simulink model "REL"  (R2022a)
settings: Solver=FixedStepDiscrete  StartTime=0.0  StopTime=10.0  FixedStep=0.01  RelTol=1e-3
libraries: simulink x4, DoorRatSts x4, DoorRlsDriver x4, DoorRlsReq x4
(part 1 of 2)
settings Model: Creator=DELL  LastModifiedBy=DELL
settings DataIOCC: SaveFormat=StructureWithTime
settings OptimizationCC: DefaultParameterBehavior=Inlined  EnhancedBackFolding=on  PassReuseOutputArgsAs=Individual arguments  ZeroExternalMemoryAtStartup=off  ZeroInternalMemoryAtStartup=off  OptimizeBlockOrder=speed  DifferentSizesBufferReuse=on  OptimizationCustomize=off  EfficientTunableParamExpr=on
settings DebuggingCC: ParameterTunabilityLossMsg=error
settings ModelReferenceCC: ModelReferenceNumInstancesAllowed=Single
settings SFSimCC: MATLABDynamicMemAlloc=off
settings RTWCC: SystemTargetFile=ert.tlc  GenCodeOnly=on  TemplateMakefile=ert_default_tmf
settings CodeAppCC: ForceParamTrailComments=on  IgnoreCustomStorageClasses=off  OperatorAnnotations=on  SimulinkDataObjDesc=on  SFDataObjDesc=on  InsertBlockDesc=on
settings ERTTargetCC: TargetLangStandard=C99 (ISO)  GenerateSampleERTMain=on  InlinedParameterPlacement=NonHierarchical  ERTCustomFileTemplate=example_file_process.tlc

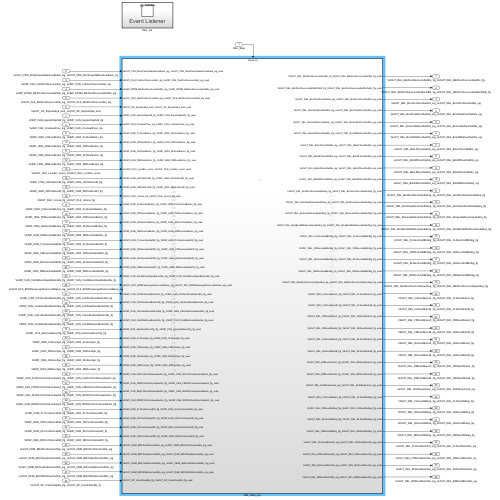
[thumbnail: Simulink's stored preview of the top-level diagram]
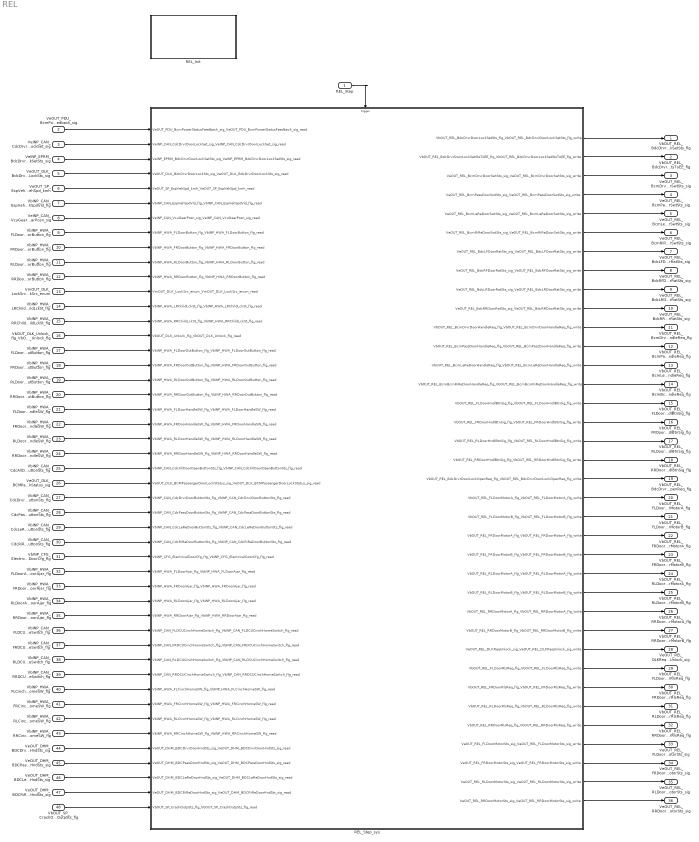
== system REL ==
  REL_Step : Inport  SampleTime=0.01  OutputFunctionCall=on
  VeOUT_PDU_BcmPowerStatusFeedback_sig_VeOUT_PDU_BcmPowerStatusFeedback_sig : Inport  Port=2  OutDataTypeStr=UInt8  PortDimensions=1
  VeINP_CAN_CdcDrvrDoorLockSet_sig_VeINP_CAN_CdcDrvrDoorLockSet_sig : Inport  Port=3  OutDataTypeStr=UInt8  PortDimensions=1
  VeINP_EPRM_BdcDrvrDoorLockSetSts_sig_VeINP_EPRM_BdcDrvrDoorLockSetSts_sig : Inport  Port=4  OutDataTypeStr=UInt8  PortDimensions=1
  VeOUT_DLK_BdcDrvrDoorLockSts_sig_VeOUT_DLK_BdcDrvrDoorLockSts_sig : Inport  Port=5  OutDataTypeStr=UInt8  PortDimensions=1
  VeOUT_SP_EspVehSpd_kmh_VeOUT_SP_EspVehSpd_kmh : Inport  Port=6  OutDataTypeStr=UInt8  PortDimensions=1
  VbINP_CAN_EspVehSpdVld_flg_VbINP_CAN_EspVehSpdVld_flg : Inport  Port=7  OutDataTypeStr=Boolean  PortDimensions=1
  VeINP_CAN_VcuGearPosn_sig_VeINP_CAN_VcuGearPosn_sig : Inport  Port=8  OutDataTypeStr=UInt8  PortDimensions=1
  VbINP_HWA_FLDoorButton_flg_VbINP_HWA_FLDoorButton_flg : Inport  Port=9  OutDataTypeStr=Boolean  PortDimensions=1
  VbINP_HWA_FRDoorButton_flg_VbINP_HWA_FRDoorButton_flg : Inport  Port=10  OutDataTypeStr=Boolean  PortDimensions=1
  VbINP_HWA_RLDoorButton_flg_VbINP_HWA_RLDoorButton_flg : Inport  Port=11  OutDataTypeStr=Boolean  PortDimensions=1
  VbINP_HWA_RRDoorButton_flg_VbINP_HWA_RRDoorButton_flg : Inport  Port=12  OutDataTypeStr=Boolean  PortDimensions=1
  VmOUT_DLK_LockSrc_enum_VmOUT_DLK_LockSrc_enum : Inport  Port=13  OutDataTypeStr=UInt8  PortDimensions=1
  VbINP_HWA_LRChildLckSt_flg_VbINP_HWA_LRChildLckSt_flg : Inport  Port=14  OutDataTypeStr=Boolean  PortDimensions=1
  VbINP_HWA_RRChildLckSt_flg_VbINP_HWA_RRChildLckSt_flg : Inport  Port=15  OutDataTypeStr=Boolean  PortDimensions=1
  VbOUT_DLK_Unlock_flg_VbOUT_DLK_Unlock_flg : Inport  Port=16  OutDataTypeStr=Boolean  PortDimensions=1
  VbINP_HWA_FLDoorOutButton_flg_VbINP_HWA_FLDoorOutButton_flg : Inport  Port=17  OutDataTypeStr=Boolean  PortDimensions=1
  VbINP_HWA_FRDoorOutButton_flg_VbINP_HWA_FRDoorOutButton_flg : Inport  Port=18  OutDataTypeStr=Boolean  PortDimensions=1
  VbINP_HWA_RLDoorOutButton_flg_VbINP_HWA_RLDoorOutButton_flg : Inport  Port=19  OutDataTypeStr=Boolean  PortDimensions=1
  VbINP_HWA_RRDoorOutButton_flg_VbINP_HWA_RRDoorOutButton_flg : Inport  Port=20  OutDataTypeStr=Boolean  PortDimensions=1
  VbINP_HWA_FLDoorHandleSW_flg_VbINP_HWA_FLDoorHandleSW_flg : Inport  Port=21  OutDataTypeStr=Boolean  PortDimensions=1
  VbINP_HWA_FRDoorHandleSW_flg_VbINP_HWA_FRDoorHandleSW_flg : Inport  Port=22  OutDataTypeStr=Boolean  PortDimensions=1
  VbINP_HWA_RLDoorHandleSW_flg_VbINP_HWA_RLDoorHandleSW_flg : Inport  Port=23  OutDataTypeStr=Boolean  PortDimensions=1
  VbINP_HWA_RRDoorHandleSW_flg_VbINP_HWA_RRDoorHandleSW_flg : Inport  Port=24  OutDataTypeStr=Boolean  PortDimensions=1
  VbINP_CAN_CdcAllDoorOpenButtonSts_flg_VbINP_CAN_CdcAllDoorOpenButtonSts_flg : Inport  Port=25  OutDataTypeStr=Boolean  PortDimensions=1
  VeOUT_DLK_BCMPassengerDoorLockStatus_sig_VeOUT_DLK_BCMPassengerDoorLockStatus_sig : Inport  Port=26  OutDataTypeStr=UInt8  PortDimensions=1
  VbINP_CAN_CdcDrvrDoorButtonSts_flg_VbINP_CAN_CdcDrvrDoorButtonSts_flg : Inport  Port=27  OutDataTypeStr=Boolean  PortDimensions=1
  VbINP_CAN_CdcPassDoorButtonSts_flg_VbINP_CAN_CdcPassDoorButtonSts_flg : Inport  Port=28  OutDataTypeStr=Boolean  PortDimensions=1
  VbINP_CAN_CdcLeReDoorButtonSts_flg_VbINP_CAN_CdcLeReDoorButtonSts_flg : Inport  Port=29  OutDataTypeStr=Boolean  PortDimensions=1
  VbINP_CAN_CdcRiReDoorButtonSts_flg_VbINP_CAN_CdcRiReDoorButtonSts_flg : Inport  Port=30  OutDataTypeStr=Boolean  PortDimensions=1
  VbINP_CFG_ElectricalDoorCfg_flg_VbINP_CFG_ElectricalDoorCfg_flg : Inport  Port=31  OutDataTypeStr=Boolean  PortDimensions=1
  VbINP_HWA_FLDoorAjar_flg_VbINP_HWA_FLDoorAjar_flg : Inport  Port=32  OutDataTypeStr=Boolean  PortDimensions=1
  VbINP_HWA_FRDoorAjar_flg_VbINP_HWA_FRDoorAjar_flg : Inport  Port=33  OutDataTypeStr=Boolean  PortDimensions=1
  VbINP_HWA_RLDoorAjar_flg_VbINP_HWA_RLDoorAjar_flg : Inport  Port=34  OutDataTypeStr=Boolean  PortDimensions=1
  VbINP_HWA_RRDoorAjar_flg_VbINP_HWA_RRDoorAjar_flg : Inport  Port=35  OutDataTypeStr=Boolean  PortDimensions=1
  VbINP_CAN_FLDCUCinchHomeSwitch_flg_VbINP_CAN_FLDCUCinchHomeSwitch_flg : Inport  Port=36  OutDataTypeStr=Boolean  PortDimensions=1
  VbINP_CAN_FRDCUCinchHomeSwitch_flg_VbINP_CAN_FRDCUCinchHomeSwitch_flg : Inport  Port=37  OutDataTypeStr=Boolean  PortDimensions=1
  VbINP_CAN_RLDCUCinchHomeSwitch_flg_VbINP_CAN_RLDCUCinchHomeSwitch_flg : Inport  Port=38  OutDataTypeStr=Boolean  PortDimensions=1
  VbINP_CAN_RRDCUCinchHomeSwitch_flg_VbINP_CAN_RRDCUCinchHomeSwitch_flg : Inport  Port=39  OutDataTypeStr=Boolean  PortDimensions=1
  VbINP_HWA_FLCinchHomeSW_flg_VbINP_HWA_FLCinchHomeSW_flg : Inport  Port=40  OutDataTypeStr=Boolean  PortDimensions=1
  VbINP_HWA_FRCinchHomeSW_flg_VbINP_HWA_FRCinchHomeSW_flg : Inport  Port=41  OutDataTypeStr=Boolean  PortDimensions=1
  VbINP_HWA_RLCinchHomeSW_flg_VbINP_HWA_RLCinchHomeSW_flg : Inport  Port=42  OutDataTypeStr=Boolean  PortDimensions=1
  VbINP_HWA_RRCinchHomeSW_flg_VbINP_HWA_RRCinchHomeSW_flg : Inport  Port=43  OutDataTypeStr=Boolean  PortDimensions=1
  VeOUT_DHM_BDCDrvrDoorHndSts_sig_VeOUT_DHM_BDCDrvrDoorHndSts_sig : Inport  Port=44  OutDataTypeStr=UInt8  PortDimensions=1
  VeOUT_DHM_BDCPassDoorHndSts_sig_VeOUT_DHM_BDCPassDoorHndSts_sig : Inport  Port=45  OutDataTypeStr=UInt8  PortDimensions=1
  VeOUT_DHM_BDCLeReDoorHndSts_sig_VeOUT_DHM_BDCLeReDoorHndSts_sig : Inport  Port=46  OutDataTypeStr=UInt8  PortDimensions=1
  VeOUT_DHM_BDCRiReDoorHndSts_sig_VeOUT_DHM_BDCRiReDoorHndSts_sig : Inport  Port=47  OutDataTypeStr=UInt8  PortDimensions=1
  VbOUT_SP_CrashOutpSts_flg_VbOUT_SP_CrashOutpSts_flg : Inport  Port=48  OutDataTypeStr=Boolean  PortDimensions=1
  REL_Init : Subsystem
  REL_Step_sys : Subsystem
  VbOUT_REL_BdcDrvrDoorLockSetSts_flg_VbOUT_REL_BdcDrvrDoorLockSetSts_flg : Outport  OutDataTypeStr=Boolean  PortDimensions=1
  VbOUT_REL_BdcDrvrDoorLockSetStsToEE_flg_VbOUT_REL_BdcDrvrDoorLockSetStsToEE_flg : Outport  Port=2  OutDataTypeStr=Boolean  PortDimensions=1
  VeOUT_REL_BcmDrvrDoorSwtSts_sig_VeOUT_REL_BcmDrvrDoorSwtSts_sig : Outport  Port=3  OutDataTypeStr=UInt8  PortDimensions=1
  VeOUT_REL_BcmPassDoorSwtSts_sig_VeOUT_REL_BcmPassDoorSwtSts_sig : Outport  Port=4  OutDataTypeStr=UInt8  PortDimensions=1
  VeOUT_REL_BcmLeReDoorSwtSts_sig_VeOUT_REL_BcmLeReDoorSwtSts_sig : Outport  Port=5  OutDataTypeStr=UInt8  PortDimensions=1
  VeOUT_REL_BcmRiReDoorSwtSts_sig_VeOUT_REL_BcmRiReDoorSwtSts_sig : Outport  Port=6  OutDataTypeStr=UInt8  PortDimensions=1
  VeOUT_REL_BdcLFDoorRatSts_sig_VeOUT_REL_BdcLFDoorRatSts_sig : Outport  Port=7  OutDataTypeStr=UInt8  PortDimensions=1
  VeOUT_REL_BdcRFDoorRatSts_sig_VeOUT_REL_BdcRFDoorRatSts_sig : Outport  Port=8  OutDataTypeStr=UInt8  PortDimensions=1
  VeOUT_REL_BdcLRDoorRatSts_sig_VeOUT_REL_BdcLRDoorRatSts_sig : Outport  Port=9  OutDataTypeStr=UInt8  PortDimensions=1
  VeOUT_REL_BdcRRDoorRatSts_sig_VeOUT_REL_BdcRRDoorRatSts_sig : Outport  Port=10  OutDataTypeStr=UInt8  PortDimensions=1
  VbOUT_REL_BcmDrvrDoorHandleReq_flg_VbOUT_REL_BcmDrvrDoorHandleReq_flg : Outport  Port=11  OutDataTypeStr=Boolean  PortDimensions=1
  VbOUT_REL_BcmPassDoorHandleReq_flg_VbOUT_REL_BcmPassDoorHandleReq_flg : Outport  Port=12  OutDataTypeStr=Boolean  PortDimensions=1
  VbOUT_REL_BcmLeReDoorHandleReq_flg_VbOUT_REL_BcmLeReDoorHandleReq_flg : Outport  Port=13  OutDataTypeStr=Boolean  PortDimensions=1
  VbOUT_REL_BcmBcmRiReDoorHandleReq_flg_VbOUT_REL_BcmBcmRiReDoorHandleReq_flg : Outport  Port=14  OutDataTypeStr=Boolean  PortDimensions=1
  VbOUT_REL_FLDoorHndlBtnSig_flg_VbOUT_REL_FLDoorHndlBtnSig_flg : Outport  Port=15  OutDataTypeStr=Boolean  PortDimensions=1
  VbOUT_REL_FRDoorHndlBtnSig_flg_VbOUT_REL_FRDoorHndlBtnSig_flg : Outport  Port=16  OutDataTypeStr=Boolean  PortDimensions=1
  VbOUT_REL_RLDoorHndlBtnSig_flg_VbOUT_REL_RLDoorHndlBtnSig_flg : Outport  Port=17  OutDataTypeStr=Boolean  PortDimensions=1
  VbOUT_REL_RRDoorHndlBtnSig_flg_VbOUT_REL_RRDoorHndlBtnSig_flg : Outport  Port=18  OutDataTypeStr=Boolean  PortDimensions=1
  VbOUT_REL_BdcDrvrDoorLockOpenReq_flg_VbOUT_REL_BdcDrvrDoorLockOpenReq_flg : Outport  Port=19  OutDataTypeStr=Boolean  PortDimensions=1
  VbOUT_REL_FLDoorMotorA_flg_VbOUT_REL_FLDoorMotorA_flg : Outport  Port=20  OutDataTypeStr=Boolean  PortDimensions=1
  VbOUT_REL_FLDoorMotorB_flg_VbOUT_REL_FLDoorMotorB_flg : Outport  Port=21  OutDataTypeStr=Boolean  PortDimensions=1
  VbOUT_REL_FRDoorMotorA_flg_VbOUT_REL_FRDoorMotorA_flg : Outport  Port=22  OutDataTypeStr=Boolean  PortDimensions=1
  VbOUT_REL_FRDoorMotorB_flg_VbOUT_REL_FRDoorMotorB_flg : Outport  Port=23  OutDataTypeStr=Boolean  PortDimensions=1
  VbOUT_REL_RLDoorMotorA_flg_VbOUT_REL_RLDoorMotorA_flg : Outport  Port=24  OutDataTypeStr=Boolean  PortDimensions=1
  VbOUT_REL_RLDoorMotorB_flg_VbOUT_REL_RLDoorMotorB_flg : Outport  Port=25  OutDataTypeStr=Boolean  PortDimensions=1
  VbOUT_REL_RRDoorMotorA_flg_VbOUT_REL_RRDoorMotorA_flg : Outport  Port=26  OutDataTypeStr=Boolean  PortDimensions=1
  VbOUT_REL_RRDoorMotorB_flg_VbOUT_REL_RRDoorMotorB_flg : Outport  Port=27  OutDataTypeStr=Boolean  PortDimensions=1
  VeOUT_REL_DLKReqUnlock_sig_VeOUT_REL_DLKReqUnlock_sig : Outport  Port=28  OutDataTypeStr=UInt8  PortDimensions=1
  VbOUT_REL_FLDoorRlsReq_flg_VbOUT_REL_FLDoorRlsReq_flg : Outport  Port=29  OutDataTypeStr=Boolean  PortDimensions=1
  VbOUT_REL_FRDoorRlsReq_flg_VbOUT_REL_FRDoorRlsReq_flg : Outport  Port=30  OutDataTypeStr=Boolean  PortDimensions=1
  VbOUT_REL_RLDoorRlsReq_flg_VbOUT_REL_RLDoorRlsReq_flg : Outport  Port=31  OutDataTypeStr=Boolean  PortDimensions=1
  VbOUT_REL_RRDoorRlsReq_flg_VbOUT_REL_RRDoorRlsReq_flg : Outport  Port=32  OutDataTypeStr=Boolean  PortDimensions=1
  VeOUT_REL_FLDoorMotorSts_sig_VeOUT_REL_FLDoorMotorSts_sig : Outport  Port=33  OutDataTypeStr=UInt8  PortDimensions=1
  VeOUT_REL_FRDoorMotorSts_sig_VeOUT_REL_FRDoorMotorSts_sig : Outport  Port=34  OutDataTypeStr=UInt8  PortDimensions=1
  VeOUT_REL_RLDoorMotorSts_sig_VeOUT_REL_RLDoorMotorSts_sig : Outport  Port=35  OutDataTypeStr=UInt8  PortDimensions=1
  VeOUT_REL_RRDoorMotorSts_sig_VeOUT_REL_RRDoorMotorSts_sig : Outport  Port=36  OutDataTypeStr=UInt8  PortDimensions=1
  wires:
  VeOUT_PDU_BcmPowerStatusFeedback_sig_VeOUT_PDU_BcmPowerStatusFeedback_sig/1 -> REL_Step_sys/1(VeOUT_PDU_BcmPowerStatusFeedback_sig_VeOUT_PDU_BcmPowerStatusFeedback_sig_read)
  VeINP_CAN_CdcDrvrDoorLockSet_sig_VeINP_CAN_CdcDrvrDoorLockSet_sig/1 -> REL_Step_sys/2(VeINP_CAN_CdcDrvrDoorLockSet_sig_VeINP_CAN_CdcDrvrDoorLockSet_sig_read)
  VeINP_EPRM_BdcDrvrDoorLockSetSts_sig_VeINP_EPRM_BdcDrvrDoorLockSetSts_sig/1 -> REL_Step_sys/3(VeINP_EPRM_BdcDrvrDoorLockSetSts_sig_VeINP_EPRM_BdcDrvrDoorLockSetSts_sig_read)
  VeOUT_DLK_BdcDrvrDoorLockSts_sig_VeOUT_DLK_BdcDrvrDoorLockSts_sig/1 -> REL_Step_sys/4(VeOUT_DLK_BdcDrvrDoorLockSts_sig_VeOUT_DLK_BdcDrvrDoorLockSts_sig_read)
  VeOUT_SP_EspVehSpd_kmh_VeOUT_SP_EspVehSpd_kmh/1 -> REL_Step_sys/5(VeOUT_SP_EspVehSpd_kmh_VeOUT_SP_EspVehSpd_kmh_read)
  VbINP_CAN_EspVehSpdVld_flg_VbINP_CAN_EspVehSpdVld_flg/1 -> REL_Step_sys/6(VbINP_CAN_EspVehSpdVld_flg_VbINP_CAN_EspVehSpdVld_flg_read)
  VeINP_CAN_VcuGearPosn_sig_VeINP_CAN_VcuGearPosn_sig/1 -> REL_Step_sys/7(VeINP_CAN_VcuGearPosn_sig_VeINP_CAN_VcuGearPosn_sig_read)
  VbINP_HWA_FLDoorButton_flg_VbINP_HWA_FLDoorButton_flg/1 -> REL_Step_sys/8(VbINP_HWA_FLDoorButton_flg_VbINP_HWA_FLDoorButton_flg_read)
  VbINP_HWA_FRDoorButton_flg_VbINP_HWA_FRDoorButton_flg/1 -> REL_Step_sys/9(VbINP_HWA_FRDoorButton_flg_VbINP_HWA_FRDoorButton_flg_read)
  VbINP_HWA_RLDoorButton_flg_VbINP_HWA_RLDoorButton_flg/1 -> REL_Step_sys/10(VbINP_HWA_RLDoorButton_flg_VbINP_HWA_RLDoorButton_flg_read)
  VbINP_HWA_RRDoorButton_flg_VbINP_HWA_RRDoorButton_flg/1 -> REL_Step_sys/11(VbINP_HWA_RRDoorButton_flg_VbINP_HWA_RRDoorButton_flg_read)
  VmOUT_DLK_LockSrc_enum_VmOUT_DLK_LockSrc_enum/1 -> REL_Step_sys/12(VmOUT_DLK_LockSrc_enum_VmOUT_DLK_LockSrc_enum_read)
  VbINP_HWA_LRChildLckSt_flg_VbINP_HWA_LRChildLckSt_flg/1 -> REL_Step_sys/13(VbINP_HWA_LRChildLckSt_flg_VbINP_HWA_LRChildLckSt_flg_read)
  VbINP_HWA_RRChildLckSt_flg_VbINP_HWA_RRChildLckSt_flg/1 -> REL_Step_sys/14(VbINP_HWA_RRChildLckSt_flg_VbINP_HWA_RRChildLckSt_flg_read)
  VbOUT_DLK_Unlock_flg_VbOUT_DLK_Unlock_flg/1 -> REL_Step_sys/15(VbOUT_DLK_Unlock_flg_VbOUT_DLK_Unlock_flg_read)
  VbINP_HWA_FLDoorOutButton_flg_VbINP_HWA_FLDoorOutButton_flg/1 -> REL_Step_sys/16(VbINP_HWA_FLDoorOutButton_flg_VbINP_HWA_FLDoorOutButton_flg_read)
  VbINP_HWA_FRDoorOutButton_flg_VbINP_HWA_FRDoorOutButton_flg/1 -> REL_Step_sys/17(VbINP_HWA_FRDoorOutButton_flg_VbINP_HWA_FRDoorOutButton_flg_read)
  VbINP_HWA_RLDoorOutButton_flg_VbINP_HWA_RLDoorOutButton_flg/1 -> REL_Step_sys/18(VbINP_HWA_RLDoorOutButton_flg_VbINP_HWA_RLDoorOutButton_flg_read)
  VbINP_HWA_RRDoorOutButton_flg_VbINP_HWA_RRDoorOutButton_flg/1 -> REL_Step_sys/19(VbINP_HWA_RRDoorOutButton_flg_VbINP_HWA_RRDoorOutButton_flg_read)
  VbINP_HWA_FLDoorHandleSW_flg_VbINP_HWA_FLDoorHandleSW_flg/1 -> REL_Step_sys/20(VbINP_HWA_FLDoorHandleSW_flg_VbINP_HWA_FLDoorHandleSW_flg_read)
  VbINP_HWA_FRDoorHandleSW_flg_VbINP_HWA_FRDoorHandleSW_flg/1 -> REL_Step_sys/21(VbINP_HWA_FRDoorHandleSW_flg_VbINP_HWA_FRDoorHandleSW_flg_read)
  VbINP_HWA_RLDoorHandleSW_flg_VbINP_HWA_RLDoorHandleSW_flg/1 -> REL_Step_sys/22(VbINP_HWA_RLDoorHandleSW_flg_VbINP_HWA_RLDoorHandleSW_flg_read)
  VbINP_HWA_RRDoorHandleSW_flg_VbINP_HWA_RRDoorHandleSW_flg/1 -> REL_Step_sys/23(VbINP_HWA_RRDoorHandleSW_flg_VbINP_HWA_RRDoorHandleSW_flg_read)
  VbINP_CAN_CdcAllDoorOpenButtonSts_flg_VbINP_CAN_CdcAllDoorOpenButtonSts_flg/1 -> REL_Step_sys/24(VbINP_CAN_CdcAllDoorOpenButtonSts_flg_VbINP_CAN_CdcAllDoorOpenButtonSts_flg_read)
  VeOUT_DLK_BCMPassengerDoorLockStatus_sig_VeOUT_DLK_BCMPassengerDoorLockStatus_sig/1 -> REL_Step_sys/25(VeOUT_DLK_BCMPassengerDoorLockStatus_sig_VeOUT_DLK_BCMPassengerDoorLockStatus_sig_read)
  VbINP_CAN_CdcDrvrDoorButtonSts_flg_VbINP_CAN_CdcDrvrDoorButtonSts_flg/1 -> REL_Step_sys/26(VbINP_CAN_CdcDrvrDoorButtonSts_flg_VbINP_CAN_CdcDrvrDoorButtonSts_flg_read)
  VbINP_CAN_CdcPassDoorButtonSts_flg_VbINP_CAN_CdcPassDoorButtonSts_flg/1 -> REL_Step_sys/27(VbINP_CAN_CdcPassDoorButtonSts_flg_VbINP_CAN_CdcPassDoorButtonSts_flg_read)
  VbINP_CAN_CdcLeReDoorButtonSts_flg_VbINP_CAN_CdcLeReDoorButtonSts_flg/1 -> REL_Step_sys/28(VbINP_CAN_CdcLeReDoorButtonSts_flg_VbINP_CAN_CdcLeReDoorButtonSts_flg_read)
  VbINP_CAN_CdcRiReDoorButtonSts_flg_VbINP_CAN_CdcRiReDoorButtonSts_flg/1 -> REL_Step_sys/29(VbINP_CAN_CdcRiReDoorButtonSts_flg_VbINP_CAN_CdcRiReDoorButtonSts_flg_read)
  VbINP_CFG_ElectricalDoorCfg_flg_VbINP_CFG_ElectricalDoorCfg_flg/1 -> REL_Step_sys/30(VbINP_CFG_ElectricalDoorCfg_flg_VbINP_CFG_ElectricalDoorCfg_flg_read)
  VbINP_HWA_FLDoorAjar_flg_VbINP_HWA_FLDoorAjar_flg/1 -> REL_Step_sys/31(VbINP_HWA_FLDoorAjar_flg_VbINP_HWA_FLDoorAjar_flg_read)
  VbINP_HWA_FRDoorAjar_flg_VbINP_HWA_FRDoorAjar_flg/1 -> REL_Step_sys/32(VbINP_HWA_FRDoorAjar_flg_VbINP_HWA_FRDoorAjar_flg_read)
  VbINP_HWA_RLDoorAjar_flg_VbINP_HWA_RLDoorAjar_flg/1 -> REL_Step_sys/33(VbINP_HWA_RLDoorAjar_flg_VbINP_HWA_RLDoorAjar_flg_read)
  VbINP_HWA_RRDoorAjar_flg_VbINP_HWA_RRDoorAjar_flg/1 -> REL_Step_sys/34(VbINP_HWA_RRDoorAjar_flg_VbINP_HWA_RRDoorAjar_flg_read)
  VbINP_CAN_FLDCUCinchHomeSwitch_flg_VbINP_CAN_FLDCUCinchHomeSwitch_flg/1 -> REL_Step_sys/35(VbINP_CAN_FLDCUCinchHomeSwitch_flg_VbINP_CAN_FLDCUCinchHomeSwitch_flg_read)
  VbINP_CAN_FRDCUCinchHomeSwitch_flg_VbINP_CAN_FRDCUCinchHomeSwitch_flg/1 -> REL_Step_sys/36(VbINP_CAN_FRDCUCinchHomeSwitch_flg_VbINP_CAN_FRDCUCinchHomeSwitch_flg_read)
  VbINP_CAN_RLDCUCinchHomeSwitch_flg_VbINP_CAN_RLDCUCinchHomeSwitch_flg/1 -> REL_Step_sys/37(VbINP_CAN_RLDCUCinchHomeSwitch_flg_VbINP_CAN_RLDCUCinchHomeSwitch_flg_read)
  VbINP_CAN_RRDCUCinchHomeSwitch_flg_VbINP_CAN_RRDCUCinchHomeSwitch_flg/1 -> REL_Step_sys/38(VbINP_CAN_RRDCUCinchHomeSwitch_flg_VbINP_CAN_RRDCUCinchHomeSwitch_flg_read)
  VbINP_HWA_FLCinchHomeSW_flg_VbINP_HWA_FLCinchHomeSW_flg/1 -> REL_Step_sys/39(VbINP_HWA_FLCinchHomeSW_flg_VbINP_HWA_FLCinchHomeSW_flg_read)
  VbINP_HWA_FRCinchHomeSW_flg_VbINP_HWA_FRCinchHomeSW_flg/1 -> REL_Step_sys/40(VbINP_HWA_FRCinchHomeSW_flg_VbINP_HWA_FRCinchHomeSW_flg_read)
  VbINP_HWA_RLCinchHomeSW_flg_VbINP_HWA_RLCinchHomeSW_flg/1 -> REL_Step_sys/41(VbINP_HWA_RLCinchHomeSW_flg_VbINP_HWA_RLCinchHomeSW_flg_read)
  VbINP_HWA_RRCinchHomeSW_flg_VbINP_HWA_RRCinchHomeSW_flg/1 -> REL_Step_sys/42(VbINP_HWA_RRCinchHomeSW_flg_VbINP_HWA_RRCinchHomeSW_flg_read)
  VeOUT_DHM_BDCDrvrDoorHndSts_sig_VeOUT_DHM_BDCDrvrDoorHndSts_sig/1 -> REL_Step_sys/43(VeOUT_DHM_BDCDrvrDoorHndSts_sig_VeOUT_DHM_BDCDrvrDoorHndSts_sig_read)
  VeOUT_DHM_BDCPassDoorHndSts_sig_VeOUT_DHM_BDCPassDoorHndSts_sig/1 -> REL_Step_sys/44(VeOUT_DHM_BDCPassDoorHndSts_sig_VeOUT_DHM_BDCPassDoorHndSts_sig_read)
  VeOUT_DHM_BDCLeReDoorHndSts_sig_VeOUT_DHM_BDCLeReDoorHndSts_sig/1 -> REL_Step_sys/45(VeOUT_DHM_BDCLeReDoorHndSts_sig_VeOUT_DHM_BDCLeReDoorHndSts_sig_read)
  VeOUT_DHM_BDCRiReDoorHndSts_sig_VeOUT_DHM_BDCRiReDoorHndSts_sig/1 -> REL_Step_sys/46(VeOUT_DHM_BDCRiReDoorHndSts_sig_VeOUT_DHM_BDCRiReDoorHndSts_sig_read)
  VbOUT_SP_CrashOutpSts_flg_VbOUT_SP_CrashOutpSts_flg/1 -> REL_Step_sys/47(VbOUT_SP_CrashOutpSts_flg_VbOUT_SP_CrashOutpSts_flg_read)
  REL_Step_sys/1(VbOUT_REL_BdcDrvrDoorLockSetSts_flg_VbOUT_REL_BdcDrvrDoorLockSetSts_flg_write) -> VbOUT_REL_BdcDrvrDoorLockSetSts_flg_VbOUT_REL_BdcDrvrDoorLockSetSts_flg/1
  REL_Step_sys/2(VbOUT_REL_BdcDrvrDoorLockSetStsToEE_flg_VbOUT_REL_BdcDrvrDoorLockSetStsToEE_flg_write) -> VbOUT_REL_BdcDrvrDoorLockSetStsToEE_flg_VbOUT_REL_BdcDrvrDoorLockSetStsToEE_flg/1
  REL_Step_sys/3(VeOUT_REL_BcmDrvrDoorSwtSts_sig_VeOUT_REL_BcmDrvrDoorSwtSts_sig_write) -> VeOUT_REL_BcmDrvrDoorSwtSts_sig_VeOUT_REL_BcmDrvrDoorSwtSts_sig/1
  REL_Step_sys/4(VeOUT_REL_BcmPassDoorSwtSts_sig_VeOUT_REL_BcmPassDoorSwtSts_sig_write) -> VeOUT_REL_BcmPassDoorSwtSts_sig_VeOUT_REL_BcmPassDoorSwtSts_sig/1
  REL_Step_sys/5(VeOUT_REL_BcmLeReDoorSwtSts_sig_VeOUT_REL_BcmLeReDoorSwtSts_sig_write) -> VeOUT_REL_BcmLeReDoorSwtSts_sig_VeOUT_REL_BcmLeReDoorSwtSts_sig/1
  REL_Step_sys/6(VeOUT_REL_BcmRiReDoorSwtSts_sig_VeOUT_REL_BcmRiReDoorSwtSts_sig_write) -> VeOUT_REL_BcmRiReDoorSwtSts_sig_VeOUT_REL_BcmRiReDoorSwtSts_sig/1
  REL_Step_sys/7(VeOUT_REL_BdcLFDoorRatSts_sig_VeOUT_REL_BdcLFDoorRatSts_sig_write) -> VeOUT_REL_BdcLFDoorRatSts_sig_VeOUT_REL_BdcLFDoorRatSts_sig/1
  REL_Step_sys/8(VeOUT_REL_BdcRFDoorRatSts_sig_VeOUT_REL_BdcRFDoorRatSts_sig_write) -> VeOUT_REL_BdcRFDoorRatSts_sig_VeOUT_REL_BdcRFDoorRatSts_sig/1
  REL_Step_sys/9(VeOUT_REL_BdcLRDoorRatSts_sig_VeOUT_REL_BdcLRDoorRatSts_sig_write) -> VeOUT_REL_BdcLRDoorRatSts_sig_VeOUT_REL_BdcLRDoorRatSts_sig/1
  REL_Step_sys/10(VeOUT_REL_BdcRRDoorRatSts_sig_VeOUT_REL_BdcRRDoorRatSts_sig_write) -> VeOUT_REL_BdcRRDoorRatSts_sig_VeOUT_REL_BdcRRDoorRatSts_sig/1
  REL_Step_sys/11(VbOUT_REL_BcmDrvrDoorHandleReq_flg_VbOUT_REL_BcmDrvrDoorHandleReq_flg_write) -> VbOUT_REL_BcmDrvrDoorHandleReq_flg_VbOUT_REL_BcmDrvrDoorHandleReq_flg/1
  REL_Step_sys/12(VbOUT_REL_BcmPassDoorHandleReq_flg_VbOUT_REL_BcmPassDoorHandleReq_flg_write) -> VbOUT_REL_BcmPassDoorHandleReq_flg_VbOUT_REL_BcmPassDoorHandleReq_flg/1
  REL_Step_sys/13(VbOUT_REL_BcmLeReDoorHandleReq_flg_VbOUT_REL_BcmLeReDoorHandleReq_flg_write) -> VbOUT_REL_BcmLeReDoorHandleReq_flg_VbOUT_REL_BcmLeReDoorHandleReq_flg/1
  REL_Step_sys/14(VbOUT_REL_BcmBcmRiReDoorHandleReq_flg_VbOUT_REL_BcmBcmRiReDoorHandleReq_flg_write) -> VbOUT_REL_BcmBcmRiReDoorHandleReq_flg_VbOUT_REL_BcmBcmRiReDoorHandleReq_flg/1
  REL_Step_sys/15(VbOUT_REL_FLDoorHndlBtnSig_flg_VbOUT_REL_FLDoorHndlBtnSig_flg_write) -> VbOUT_REL_FLDoorHndlBtnSig_flg_VbOUT_REL_FLDoorHndlBtnSig_flg/1
  REL_Step_sys/16(VbOUT_REL_FRDoorHndlBtnSig_flg_VbOUT_REL_FRDoorHndlBtnSig_flg_write) -> VbOUT_REL_FRDoorHndlBtnSig_flg_VbOUT_REL_FRDoorHndlBtnSig_flg/1
  REL_Step_sys/17(VbOUT_REL_RLDoorHndlBtnSig_flg_VbOUT_REL_RLDoorHndlBtnSig_flg_write) -> VbOUT_REL_RLDoorHndlBtnSig_flg_VbOUT_REL_RLDoorHndlBtnSig_flg/1
  REL_Step_sys/18(VbOUT_REL_RRDoorHndlBtnSig_flg_VbOUT_REL_RRDoorHndlBtnSig_flg_write) -> VbOUT_REL_RRDoorHndlBtnSig_flg_VbOUT_REL_RRDoorHndlBtnSig_flg/1
  REL_Step_sys/19(VbOUT_REL_BdcDrvrDoorLockOpenReq_flg_VbOUT_REL_BdcDrvrDoorLockOpenReq_flg_write) -> VbOUT_REL_BdcDrvrDoorLockOpenReq_flg_VbOUT_REL_BdcDrvrDoorLockOpenReq_flg/1
  REL_Step_sys/20(VbOUT_REL_FLDoorMotorA_flg_VbOUT_REL_FLDoorMotorA_flg_write) -> VbOUT_REL_FLDoorMotorA_flg_VbOUT_REL_FLDoorMotorA_flg/1
  REL_Step_sys/21(VbOUT_REL_FLDoorMotorB_flg_VbOUT_REL_FLDoorMotorB_flg_write) -> VbOUT_REL_FLDoorMotorB_flg_VbOUT_REL_FLDoorMotorB_flg/1
  REL_Step_sys/22(VbOUT_REL_FRDoorMotorA_flg_VbOUT_REL_FRDoorMotorA_flg_write) -> VbOUT_REL_FRDoorMotorA_flg_VbOUT_REL_FRDoorMotorA_flg/1
  REL_Step_sys/23(VbOUT_REL_FRDoorMotorB_flg_VbOUT_REL_FRDoorMotorB_flg_write) -> VbOUT_REL_FRDoorMotorB_flg_VbOUT_REL_FRDoorMotorB_flg/1
  REL_Step_sys/24(VbOUT_REL_RLDoorMotorA_flg_VbOUT_REL_RLDoorMotorA_flg_write) -> VbOUT_REL_RLDoorMotorA_flg_VbOUT_REL_RLDoorMotorA_flg/1
  REL_Step_sys/25(VbOUT_REL_RLDoorMotorB_flg_VbOUT_REL_RLDoorMotorB_flg_write) -> VbOUT_REL_RLDoorMotorB_flg_VbOUT_REL_RLDoorMotorB_flg/1
  REL_Step_sys/26(VbOUT_REL_RRDoorMotorA_flg_VbOUT_REL_RRDoorMotorA_flg_write) -> VbOUT_REL_RRDoorMotorA_flg_VbOUT_REL_RRDoorMotorA_flg/1
  REL_Step_sys/27(VbOUT_REL_RRDoorMotorB_flg_VbOUT_REL_RRDoorMotorB_flg_write) -> VbOUT_REL_RRDoorMotorB_flg_VbOUT_REL_RRDoorMotorB_flg/1
  REL_Step_sys/28(VeOUT_REL_DLKReqUnlock_sig_VeOUT_REL_DLKReqUnlock_sig_write) -> VeOUT_REL_DLKReqUnlock_sig_VeOUT_REL_DLKReqUnlock_sig/1
  REL_Step_sys/29(VbOUT_REL_FLDoorRlsReq_flg_VbOUT_REL_FLDoorRlsReq_flg_write) -> VbOUT_REL_FLDoorRlsReq_flg_VbOUT_REL_FLDoorRlsReq_flg/1
  REL_Step_sys/30(VbOUT_REL_FRDoorRlsReq_flg_VbOUT_REL_FRDoorRlsReq_flg_write) -> VbOUT_REL_FRDoorRlsReq_flg_VbOUT_REL_FRDoorRlsReq_flg/1
  REL_Step_sys/31(VbOUT_REL_RLDoorRlsReq_flg_VbOUT_REL_RLDoorRlsReq_flg_write) -> VbOUT_REL_RLDoorRlsReq_flg_VbOUT_REL_RLDoorRlsReq_flg/1
  REL_Step_sys/32(VbOUT_REL_RRDoorRlsReq_flg_VbOUT_REL_RRDoorRlsReq_flg_write) -> VbOUT_REL_RRDoorRlsReq_flg_VbOUT_REL_RRDoorRlsReq_flg/1
  REL_Step_sys/33(VeOUT_REL_FLDoorMotorSts_sig_VeOUT_REL_FLDoorMotorSts_sig_write) -> VeOUT_REL_FLDoorMotorSts_sig_VeOUT_REL_FLDoorMotorSts_sig/1
  REL_Step_sys/34(VeOUT_REL_FRDoorMotorSts_sig_VeOUT_REL_FRDoorMotorSts_sig_write) -> VeOUT_REL_FRDoorMotorSts_sig_VeOUT_REL_FRDoorMotorSts_sig/1
  REL_Step_sys/35(VeOUT_REL_RLDoorMotorSts_sig_VeOUT_REL_RLDoorMotorSts_sig_write) -> VeOUT_REL_RLDoorMotorSts_sig_VeOUT_REL_RLDoorMotorSts_sig/1
  REL_Step_sys/36(VeOUT_REL_RRDoorMotorSts_sig_VeOUT_REL_RRDoorMotorSts_sig_write) -> VeOUT_REL_RRDoorMotorSts_sig_VeOUT_REL_RRDoorMotorSts_sig/1
  REL_Step/1 -> REL_Step_sys/Trigger

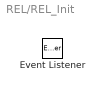
== system REL/REL_Init ==
  Event Listener : EventListener  EventName=reset

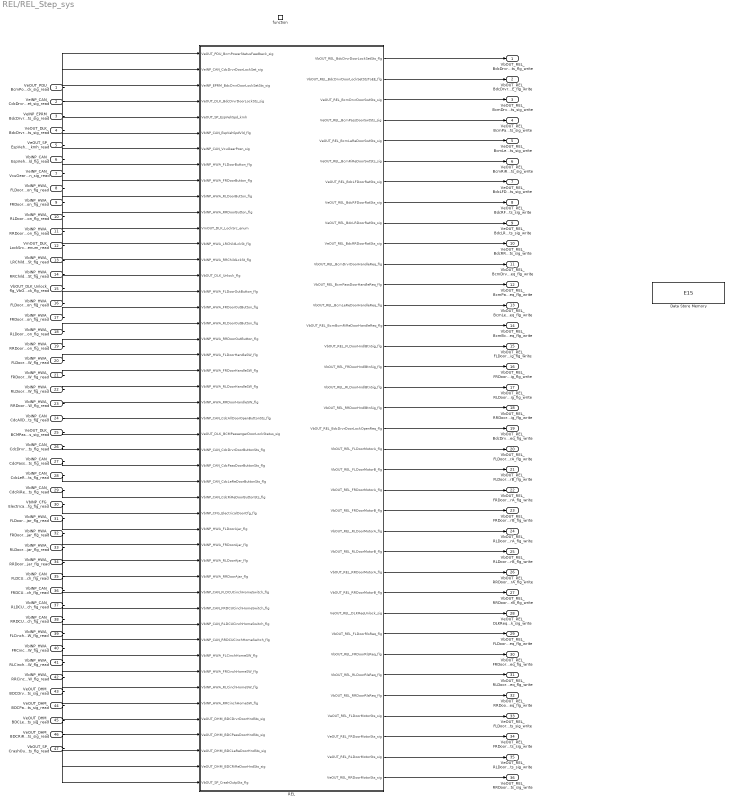
== system REL/REL_Step_sys ==
  VeOUT_PDU_BcmPowerStatusFeedback_sig_VeOUT_PDU_BcmPowerStatusFeedback_sig_read : Inport
  VeINP_CAN_CdcDrvrDoorLockSet_sig_VeINP_CAN_CdcDrvrDoorLockSet_sig_read : Inport  Port=2
  VeINP_EPRM_BdcDrvrDoorLockSetSts_sig_VeINP_EPRM_BdcDrvrDoorLockSetSts_sig_read : Inport  Port=3
  VeOUT_DLK_BdcDrvrDoorLockSts_sig_VeOUT_DLK_BdcDrvrDoorLockSts_sig_read : Inport  Port=4
  VeOUT_SP_EspVehSpd_kmh_VeOUT_SP_EspVehSpd_kmh_read : Inport  Port=5
  VbINP_CAN_EspVehSpdVld_flg_VbINP_CAN_EspVehSpdVld_flg_read : Inport  Port=6
  VeINP_CAN_VcuGearPosn_sig_VeINP_CAN_VcuGearPosn_sig_read : Inport  Port=7
  VbINP_HWA_FLDoorButton_flg_VbINP_HWA_FLDoorButton_flg_read : Inport  Port=8
  VbINP_HWA_FRDoorButton_flg_VbINP_HWA_FRDoorButton_flg_read : Inport  Port=9
  VbINP_HWA_RLDoorButton_flg_VbINP_HWA_RLDoorButton_flg_read : Inport  Port=10
  VbINP_HWA_RRDoorButton_flg_VbINP_HWA_RRDoorButton_flg_read : Inport  Port=11
  VmOUT_DLK_LockSrc_enum_VmOUT_DLK_LockSrc_enum_read : Inport  Port=12
  VbINP_HWA_LRChildLckSt_flg_VbINP_HWA_LRChildLckSt_flg_read : Inport  Port=13
  VbINP_HWA_RRChildLckSt_flg_VbINP_HWA_RRChildLckSt_flg_read : Inport  Port=14
  VbOUT_DLK_Unlock_flg_VbOUT_DLK_Unlock_flg_read : Inport  Port=15
  VbINP_HWA_FLDoorOutButton_flg_VbINP_HWA_FLDoorOutButton_flg_read : Inport  Port=16
  VbINP_HWA_FRDoorOutButton_flg_VbINP_HWA_FRDoorOutButton_flg_read : Inport  Port=17
  VbINP_HWA_RLDoorOutButton_flg_VbINP_HWA_RLDoorOutButton_flg_read : Inport  Port=18
  VbINP_HWA_RRDoorOutButton_flg_VbINP_HWA_RRDoorOutButton_flg_read : Inport  Port=19
  VbINP_HWA_FLDoorHandleSW_flg_VbINP_HWA_FLDoorHandleSW_flg_read : Inport  Port=20
  VbINP_HWA_FRDoorHandleSW_flg_VbINP_HWA_FRDoorHandleSW_flg_read : Inport  Port=21
  VbINP_HWA_RLDoorHandleSW_flg_VbINP_HWA_RLDoorHandleSW_flg_read : Inport  Port=22
  VbINP_HWA_RRDoorHandleSW_flg_VbINP_HWA_RRDoorHandleSW_flg_read : Inport  Port=23
  VbINP_CAN_CdcAllDoorOpenButtonSts_flg_VbINP_CAN_CdcAllDoorOpenButtonSts_flg_read : Inport  Port=24
  VeOUT_DLK_BCMPassengerDoorLockStatus_sig_VeOUT_DLK_BCMPassengerDoorLockStatus_sig_read : Inport  Port=25
  VbINP_CAN_CdcDrvrDoorButtonSts_flg_VbINP_CAN_CdcDrvrDoorButtonSts_flg_read : Inport  Port=26
  VbINP_CAN_CdcPassDoorButtonSts_flg_VbINP_CAN_CdcPassDoorButtonSts_flg_read : Inport  Port=27
  VbINP_CAN_CdcLeReDoorButtonSts_flg_VbINP_CAN_CdcLeReDoorButtonSts_flg_read : Inport  Port=28
  VbINP_CAN_CdcRiReDoorButtonSts_flg_VbINP_CAN_CdcRiReDoorButtonSts_flg_read : Inport  Port=29
  VbINP_CFG_ElectricalDoorCfg_flg_VbINP_CFG_ElectricalDoorCfg_flg_read : Inport  Port=30
  VbINP_HWA_FLDoorAjar_flg_VbINP_HWA_FLDoorAjar_flg_read : Inport  Port=31
  VbINP_HWA_FRDoorAjar_flg_VbINP_HWA_FRDoorAjar_flg_read : Inport  Port=32
  VbINP_HWA_RLDoorAjar_flg_VbINP_HWA_RLDoorAjar_flg_read : Inport  Port=33
  VbINP_HWA_RRDoorAjar_flg_VbINP_HWA_RRDoorAjar_flg_read : Inport  Port=34
  VbINP_CAN_FLDCUCinchHomeSwitch_flg_VbINP_CAN_FLDCUCinchHomeSwitch_flg_read : Inport  Port=35
  VbINP_CAN_FRDCUCinchHomeSwitch_flg_VbINP_CAN_FRDCUCinchHomeSwitch_flg_read : Inport  Port=36
  VbINP_CAN_RLDCUCinchHomeSwitch_flg_VbINP_CAN_RLDCUCinchHomeSwitch_flg_read : Inport  Port=37
  VbINP_CAN_RRDCUCinchHomeSwitch_flg_VbINP_CAN_RRDCUCinchHomeSwitch_flg_read : Inport  Port=38
  VbINP_HWA_FLCinchHomeSW_flg_VbINP_HWA_FLCinchHomeSW_flg_read : Inport  Port=39
  VbINP_HWA_FRCinchHomeSW_flg_VbINP_HWA_FRCinchHomeSW_flg_read : Inport  Port=40
  VbINP_HWA_RLCinchHomeSW_flg_VbINP_HWA_RLCinchHomeSW_flg_read : Inport  Port=41
  VbINP_HWA_RRCinchHomeSW_flg_VbINP_HWA_RRCinchHomeSW_flg_read : Inport  Port=42
  VeOUT_DHM_BDCDrvrDoorHndSts_sig_VeOUT_DHM_BDCDrvrDoorHndSts_sig_read : Inport  Port=43
  VeOUT_DHM_BDCPassDoorHndSts_sig_VeOUT_DHM_BDCPassDoorHndSts_sig_read : Inport  Port=44
  VeOUT_DHM_BDCLeReDoorHndSts_sig_VeOUT_DHM_BDCLeReDoorHndSts_sig_read : Inport  Port=45
  VeOUT_DHM_BDCRiReDoorHndSts_sig_VeOUT_DHM_BDCRiReDoorHndSts_sig_read : Inport  Port=46
  VbOUT_SP_CrashOutpSts_flg_VbOUT_SP_CrashOutpSts_flg_read : Inport  Port=47
  function : TriggerPort  TriggerType=function-call  VariantControl=(inherit)  SampleTimeType=periodic  SampleTime=-1
  Data Store Memory : DataStoreMemory  DataStoreName=E15  WriteAfterWriteMsg=warning  ShowAdditionalParam=off
  REL : Subsystem
  VbOUT_REL_BdcDrvrDoorLockSetSts_flg_VbOUT_REL_BdcDrvrDoorLockSetSts_flg_write : Outport
      settings: EnsureOutportIsVirtual=on
  VbOUT_REL_BdcDrvrDoorLockSetStsToEE_flg_VbOUT_REL_BdcDrvrDoorLockSetStsToEE_flg_write : Outport  Port=2
      settings: EnsureOutportIsVirtual=on
  VeOUT_REL_BcmDrvrDoorSwtSts_sig_VeOUT_REL_BcmDrvrDoorSwtSts_sig_write : Outport  Port=3
      settings: EnsureOutportIsVirtual=on
  VeOUT_REL_BcmPassDoorSwtSts_sig_VeOUT_REL_BcmPassDoorSwtSts_sig_write : Outport  Port=4
      settings: EnsureOutportIsVirtual=on
  VeOUT_REL_BcmLeReDoorSwtSts_sig_VeOUT_REL_BcmLeReDoorSwtSts_sig_write : Outport  Port=5
      settings: EnsureOutportIsVirtual=on
  VeOUT_REL_BcmRiReDoorSwtSts_sig_VeOUT_REL_BcmRiReDoorSwtSts_sig_write : Outport  Port=6
      settings: EnsureOutportIsVirtual=on
  VeOUT_REL_BdcLFDoorRatSts_sig_VeOUT_REL_BdcLFDoorRatSts_sig_write : Outport  Port=7
      settings: EnsureOutportIsVirtual=on
  VeOUT_REL_BdcRFDoorRatSts_sig_VeOUT_REL_BdcRFDoorRatSts_sig_write : Outport  Port=8
      settings: EnsureOutportIsVirtual=on
  VeOUT_REL_BdcLRDoorRatSts_sig_VeOUT_REL_BdcLRDoorRatSts_sig_write : Outport  Port=9
      settings: EnsureOutportIsVirtual=on
  VeOUT_REL_BdcRRDoorRatSts_sig_VeOUT_REL_BdcRRDoorRatSts_sig_write : Outport  Port=10
      settings: EnsureOutportIsVirtual=on
  VbOUT_REL_BcmDrvrDoorHandleReq_flg_VbOUT_REL_BcmDrvrDoorHandleReq_flg_write : Outport  Port=11
      settings: EnsureOutportIsVirtual=on
  VbOUT_REL_BcmPassDoorHandleReq_flg_VbOUT_REL_BcmPassDoorHandleReq_flg_write : Outport  Port=12
      settings: EnsureOutportIsVirtual=on
  VbOUT_REL_BcmLeReDoorHandleReq_flg_VbOUT_REL_BcmLeReDoorHandleReq_flg_write : Outport  Port=13
      settings: EnsureOutportIsVirtual=on
  VbOUT_REL_BcmBcmRiReDoorHandleReq_flg_VbOUT_REL_BcmBcmRiReDoorHandleReq_flg_write : Outport  Port=14
      settings: EnsureOutportIsVirtual=on
  VbOUT_REL_FLDoorHndlBtnSig_flg_VbOUT_REL_FLDoorHndlBtnSig_flg_write : Outport  Port=15
      settings: EnsureOutportIsVirtual=on
  VbOUT_REL_FRDoorHndlBtnSig_flg_VbOUT_REL_FRDoorHndlBtnSig_flg_write : Outport  Port=16
      settings: EnsureOutportIsVirtual=on
  VbOUT_REL_RLDoorHndlBtnSig_flg_VbOUT_REL_RLDoorHndlBtnSig_flg_write : Outport  Port=17
      settings: EnsureOutportIsVirtual=on
  VbOUT_REL_RRDoorHndlBtnSig_flg_VbOUT_REL_RRDoorHndlBtnSig_flg_write : Outport  Port=18
      settings: EnsureOutportIsVirtual=on
  VbOUT_REL_BdcDrvrDoorLockOpenReq_flg_VbOUT_REL_BdcDrvrDoorLockOpenReq_flg_write : Outport  Port=19
      settings: EnsureOutportIsVirtual=on
  VbOUT_REL_FLDoorMotorA_flg_VbOUT_REL_FLDoorMotorA_flg_write : Outport  Port=20
      settings: EnsureOutportIsVirtual=on
  VbOUT_REL_FLDoorMotorB_flg_VbOUT_REL_FLDoorMotorB_flg_write : Outport  Port=21
      settings: EnsureOutportIsVirtual=on
  VbOUT_REL_FRDoorMotorA_flg_VbOUT_REL_FRDoorMotorA_flg_write : Outport  Port=22
      settings: EnsureOutportIsVirtual=on
  VbOUT_REL_FRDoorMotorB_flg_VbOUT_REL_FRDoorMotorB_flg_write : Outport  Port=23
      settings: EnsureOutportIsVirtual=on
  VbOUT_REL_RLDoorMotorA_flg_VbOUT_REL_RLDoorMotorA_flg_write : Outport  Port=24
      settings: EnsureOutportIsVirtual=on
  VbOUT_REL_RLDoorMotorB_flg_VbOUT_REL_RLDoorMotorB_flg_write : Outport  Port=25
      settings: EnsureOutportIsVirtual=on
  VbOUT_REL_RRDoorMotorA_flg_VbOUT_REL_RRDoorMotorA_flg_write : Outport  Port=26
      settings: EnsureOutportIsVirtual=on
  VbOUT_REL_RRDoorMotorB_flg_VbOUT_REL_RRDoorMotorB_flg_write : Outport  Port=27
      settings: EnsureOutportIsVirtual=on
  VeOUT_REL_DLKReqUnlock_sig_VeOUT_REL_DLKReqUnlock_sig_write : Outport  Port=28
      settings: EnsureOutportIsVirtual=on
  VbOUT_REL_FLDoorRlsReq_flg_VbOUT_REL_FLDoorRlsReq_flg_write : Outport  Port=29
      settings: EnsureOutportIsVirtual=on
  VbOUT_REL_FRDoorRlsReq_flg_VbOUT_REL_FRDoorRlsReq_flg_write : Outport  Port=30
      settings: EnsureOutportIsVirtual=on
  VbOUT_REL_RLDoorRlsReq_flg_VbOUT_REL_RLDoorRlsReq_flg_write : Outport  Port=31
      settings: EnsureOutportIsVirtual=on
  VbOUT_REL_RRDoorRlsReq_flg_VbOUT_REL_RRDoorRlsReq_flg_write : Outport  Port=32
      settings: EnsureOutportIsVirtual=on
  VeOUT_REL_FLDoorMotorSts_sig_VeOUT_REL_FLDoorMotorSts_sig_write : Outport  Port=33
      settings: EnsureOutportIsVirtual=on
  VeOUT_REL_FRDoorMotorSts_sig_VeOUT_REL_FRDoorMotorSts_sig_write : Outport  Port=34
      settings: EnsureOutportIsVirtual=on
  VeOUT_REL_RLDoorMotorSts_sig_VeOUT_REL_RLDoorMotorSts_sig_write : Outport  Port=35
      settings: EnsureOutportIsVirtual=on
  VeOUT_REL_RRDoorMotorSts_sig_VeOUT_REL_RRDoorMotorSts_sig_write : Outport  Port=36
      settings: EnsureOutportIsVirtual=on
  wires:
  REL/1(VbOUT_REL_BdcDrvrDoorLockSetSts_flg) -> VbOUT_REL_BdcDrvrDoorLockSetSts_flg_VbOUT_REL_BdcDrvrDoorLockSetSts_flg_write/1
  REL/2(VbOUT_REL_BdcDrvrDoorLockSetStsToEE_flg) -> VbOUT_REL_BdcDrvrDoorLockSetStsToEE_flg_VbOUT_REL_BdcDrvrDoorLockSetStsToEE_flg_write/1
  REL/3(VeOUT_REL_BcmDrvrDoorSwtSts_sig) -> VeOUT_REL_BcmDrvrDoorSwtSts_sig_VeOUT_REL_BcmDrvrDoorSwtSts_sig_write/1
  REL/4(VeOUT_REL_BcmPassDoorSwtSts_sig) -> VeOUT_REL_BcmPassDoorSwtSts_sig_VeOUT_REL_BcmPassDoorSwtSts_sig_write/1
  REL/5(VeOUT_REL_BcmLeReDoorSwtSts_sig) -> VeOUT_REL_BcmLeReDoorSwtSts_sig_VeOUT_REL_BcmLeReDoorSwtSts_sig_write/1
  REL/6(VeOUT_REL_BcmRiReDoorSwtSts_sig) -> VeOUT_REL_BcmRiReDoorSwtSts_sig_VeOUT_REL_BcmRiReDoorSwtSts_sig_write/1
  REL/7(VeOUT_REL_BdcLFDoorRatSts_sig) -> VeOUT_REL_BdcLFDoorRatSts_sig_VeOUT_REL_BdcLFDoorRatSts_sig_write/1
  REL/8(VeOUT_REL_BdcRFDoorRatSts_sig) -> VeOUT_REL_BdcRFDoorRatSts_sig_VeOUT_REL_BdcRFDoorRatSts_sig_write/1
  REL/9(VeOUT_REL_BdcLRDoorRatSts_sig) -> VeOUT_REL_BdcLRDoorRatSts_sig_VeOUT_REL_BdcLRDoorRatSts_sig_write/1
  REL/10(VeOUT_REL_BdcRRDoorRatSts_sig) -> VeOUT_REL_BdcRRDoorRatSts_sig_VeOUT_REL_BdcRRDoorRatSts_sig_write/1
  REL/11(VbOUT_REL_BcmDrvrDoorHandleReq_flg) -> VbOUT_REL_BcmDrvrDoorHandleReq_flg_VbOUT_REL_BcmDrvrDoorHandleReq_flg_write/1
  REL/12(VbOUT_REL_BcmPassDoorHandleReq_flg) -> VbOUT_REL_BcmPassDoorHandleReq_flg_VbOUT_REL_BcmPassDoorHandleReq_flg_write/1
  REL/13(VbOUT_REL_BcmLeReDoorHandleReq_flg) -> VbOUT_REL_BcmLeReDoorHandleReq_flg_VbOUT_REL_BcmLeReDoorHandleReq_flg_write/1
  REL/14(VbOUT_REL_BcmBcmRiReDoorHandleReq_flg) -> VbOUT_REL_BcmBcmRiReDoorHandleReq_flg_VbOUT_REL_BcmBcmRiReDoorHandleReq_flg_write/1
  REL/15(VbOUT_REL_FLDoorHndlBtnSig_flg) -> VbOUT_REL_FLDoorHndlBtnSig_flg_VbOUT_REL_FLDoorHndlBtnSig_flg_write/1
  REL/16(VbOUT_REL_FRDoorHndlBtnSig_flg) -> VbOUT_REL_FRDoorHndlBtnSig_flg_VbOUT_REL_FRDoorHndlBtnSig_flg_write/1
  REL/17(VbOUT_REL_RLDoorHndlBtnSig_flg) -> VbOUT_REL_RLDoorHndlBtnSig_flg_VbOUT_REL_RLDoorHndlBtnSig_flg_write/1
  REL/18(VbOUT_REL_RRDoorHndlBtnSig_flg) -> VbOUT_REL_RRDoorHndlBtnSig_flg_VbOUT_REL_RRDoorHndlBtnSig_flg_write/1
  REL/19(VbOUT_REL_BdcDrvrDoorLockOpenReq_flg) -> VbOUT_REL_BdcDrvrDoorLockOpenReq_flg_VbOUT_REL_BdcDrvrDoorLockOpenReq_flg_write/1
  REL/20(VbOUT_REL_FLDoorMotorA_flg) -> VbOUT_REL_FLDoorMotorA_flg_VbOUT_REL_FLDoorMotorA_flg_write/1
  REL/21(VbOUT_REL_FLDoorMotorB_flg) -> VbOUT_REL_FLDoorMotorB_flg_VbOUT_REL_FLDoorMotorB_flg_write/1
  REL/22(VbOUT_REL_FRDoorMotorA_flg) -> VbOUT_REL_FRDoorMotorA_flg_VbOUT_REL_FRDoorMotorA_flg_write/1
  REL/23(VbOUT_REL_FRDoorMotorB_flg) -> VbOUT_REL_FRDoorMotorB_flg_VbOUT_REL_FRDoorMotorB_flg_write/1
  REL/24(VbOUT_REL_RLDoorMotorA_flg) -> VbOUT_REL_RLDoorMotorA_flg_VbOUT_REL_RLDoorMotorA_flg_write/1
  REL/25(VbOUT_REL_RLDoorMotorB_flg) -> VbOUT_REL_RLDoorMotorB_flg_VbOUT_REL_RLDoorMotorB_flg_write/1
  REL/26(VbOUT_REL_RRDoorMotorA_flg) -> VbOUT_REL_RRDoorMotorA_flg_VbOUT_REL_RRDoorMotorA_flg_write/1
  REL/27(VbOUT_REL_RRDoorMotorB_flg) -> VbOUT_REL_RRDoorMotorB_flg_VbOUT_REL_RRDoorMotorB_flg_write/1
  REL/28(VeOUT_REL_DLKReqUnlock_sig) -> VeOUT_REL_DLKReqUnlock_sig_VeOUT_REL_DLKReqUnlock_sig_write/1
  REL/29(VbOUT_REL_FLDoorRlsReq_flg) -> VbOUT_REL_FLDoorRlsReq_flg_VbOUT_REL_FLDoorRlsReq_flg_write/1
  REL/30(VbOUT_REL_FRDoorRlsReq_flg) -> VbOUT_REL_FRDoorRlsReq_flg_VbOUT_REL_FRDoorRlsReq_flg_write/1
  REL/31(VbOUT_REL_RLDoorRlsReq_flg) -> VbOUT_REL_RLDoorRlsReq_flg_VbOUT_REL_RLDoorRlsReq_flg_write/1
  REL/32(VbOUT_REL_RRDoorRlsReq_flg) -> VbOUT_REL_RRDoorRlsReq_flg_VbOUT_REL_RRDoorRlsReq_flg_write/1
  REL/33(VeOUT_REL_FLDoorMotorSts_sig) -> VeOUT_REL_FLDoorMotorSts_sig_VeOUT_REL_FLDoorMotorSts_sig_write/1
  REL/34(VeOUT_REL_FRDoorMotorSts_sig) -> VeOUT_REL_FRDoorMotorSts_sig_VeOUT_REL_FRDoorMotorSts_sig_write/1
  REL/35(VeOUT_REL_RLDoorMotorSts_sig) -> VeOUT_REL_RLDoorMotorSts_sig_VeOUT_REL_RLDoorMotorSts_sig_write/1
  REL/36(VeOUT_REL_RRDoorMotorSts_sig) -> VeOUT_REL_RRDoorMotorSts_sig_VeOUT_REL_RRDoorMotorSts_sig_write/1
  VbINP_CFG_ElectricalDoorCfg_flg_VbINP_CFG_ElectricalDoorCfg_flg_read/1 -> REL/30(VbINP_CFG_ElectricalDoorCfg_flg)
  VbINP_HWA_FLDoorAjar_flg_VbINP_HWA_FLDoorAjar_flg_read/1 -> REL/31(VbINP_HWA_FLDoorAjar_flg)
  VbINP_CAN_CdcLeReDoorButtonSts_flg_VbINP_CAN_CdcLeReDoorButtonSts_flg_read/1 -> REL/28(VbINP_CAN_CdcLeReDoorButtonSts_flg)
  VbINP_CAN_CdcRiReDoorButtonSts_flg_VbINP_CAN_CdcRiReDoorButtonSts_flg_read/1 -> REL/29(VbINP_CAN_CdcRiReDoorButtonSts_flg)
  VbINP_HWA_FRDoorAjar_flg_VbINP_HWA_FRDoorAjar_flg_read/1 -> REL/32(VbINP_HWA_FRDoorAjar_flg)
  VbINP_CAN_CdcPassDoorButtonSts_flg_VbINP_CAN_CdcPassDoorButtonSts_flg_read/1 -> REL/27(VbINP_CAN_CdcPassDoorButtonSts_flg)
  VbINP_HWA_RLDoorAjar_flg_VbINP_HWA_RLDoorAjar_flg_read/1 -> REL/33(VbINP_HWA_RLDoorAjar_flg)
  VbINP_HWA_RRDoorAjar_flg_VbINP_HWA_RRDoorAjar_flg_read/1 -> REL/34(VbINP_HWA_RRDoorAjar_flg)
  VeOUT_DLK_BCMPassengerDoorLockStatus_sig_VeOUT_DLK_BCMPassengerDoorLockStatus_sig_read/1 -> REL/25(VeOUT_DLK_BCMPassengerDoorLockStatus_sig)
  VbINP_CAN_CdcDrvrDoorButtonSts_flg_VbINP_CAN_CdcDrvrDoorButtonSts_flg_read/1 -> REL/26(VbINP_CAN_CdcDrvrDoorButtonSts_flg)
  VbINP_CAN_FLDCUCinchHomeSwitch_flg_VbINP_CAN_FLDCUCinchHomeSwitch_flg_read/1 -> REL/35(VbINP_CAN_FLDCUCinchHomeSwitch_flg)
  VbINP_CAN_FRDCUCinchHomeSwitch_flg_VbINP_CAN_FRDCUCinchHomeSwitch_flg_read/1 -> REL/36(VbINP_CAN_FRDCUCinchHomeSwitch_flg)
  VbINP_HWA_RRDoorHandleSW_flg_VbINP_HWA_RRDoorHandleSW_flg_read/1 -> REL/23(VbINP_HWA_RRDoorHandleSW_flg)
  VbINP_CAN_CdcAllDoorOpenButtonSts_flg_VbINP_CAN_CdcAllDoorOpenButtonSts_flg_read/1 -> REL/24(VbINP_CAN_CdcAllDoorOpenButtonSts_flg)
  VbINP_CAN_RLDCUCinchHomeSwitch_flg_VbINP_CAN_RLDCUCinchHomeSwitch_flg_read/1 -> REL/37(VbINP_CAN_RLDCUCinchHomeSwitch_flg)
  VbINP_HWA_RLDoorHandleSW_flg_VbINP_HWA_RLDoorHandleSW_flg_read/1 -> REL/22(VbINP_HWA_RLDoorHandleSW_flg)
  VbINP_CAN_RRDCUCinchHomeSwitch_flg_VbINP_CAN_RRDCUCinchHomeSwitch_flg_read/1 -> REL/38(VbINP_CAN_RRDCUCinchHomeSwitch_flg)
  VbINP_HWA_FLCinchHomeSW_flg_VbINP_HWA_FLCinchHomeSW_flg_read/1 -> REL/39(VbINP_HWA_FLCinchHomeSW_flg)
  VbINP_HWA_FLDoorHandleSW_flg_VbINP_HWA_FLDoorHandleSW_flg_read/1 -> REL/20(VbINP_HWA_FLDoorHandleSW_flg)
  VbINP_HWA_FRDoorHandleSW_flg_VbINP_HWA_FRDoorHandleSW_flg_read/1 -> REL/21(VbINP_HWA_FRDoorHandleSW_flg)
  VbINP_HWA_FRCinchHomeSW_flg_VbINP_HWA_FRCinchHomeSW_flg_read/1 -> REL/40(VbINP_HWA_FRCinchHomeSW_flg)
  VbINP_HWA_RLCinchHomeSW_flg_VbINP_HWA_RLCinchHomeSW_flg_read/1 -> REL/41(VbINP_HWA_RLCinchHomeSW_flg)
  VbINP_HWA_RLDoorOutButton_flg_VbINP_HWA_RLDoorOutButton_flg_read/1 -> REL/18(VbINP_HWA_RLDoorOutButton_flg)
  VbINP_HWA_RRDoorOutButton_flg_VbINP_HWA_RRDoorOutButton_flg_read/1 -> REL/19(VbINP_HWA_RRDoorOutButton_flg)
  VbINP_HWA_RRCinchHomeSW_flg_VbINP_HWA_RRCinchHomeSW_flg_read/1 -> REL/42(VbINP_HWA_RRCinchHomeSW_flg)
  VbINP_HWA_FRDoorOutButton_flg_VbINP_HWA_FRDoorOutButton_flg_read/1 -> REL/17(VbINP_HWA_FRDoorOutButton_flg)
  VeOUT_DHM_BDCDrvrDoorHndSts_sig_VeOUT_DHM_BDCDrvrDoorHndSts_sig_read/1 -> REL/43(VeOUT_DHM_BDCDrvrDoorHndSts_sig)
  VeOUT_DHM_BDCPassDoorHndSts_sig_VeOUT_DHM_BDCPassDoorHndSts_sig_read/1 -> REL/44(VeOUT_DHM_BDCPassDoorHndSts_sig)
  VbOUT_DLK_Unlock_flg_VbOUT_DLK_Unlock_flg_read/1 -> REL/15(VbOUT_DLK_Unlock_flg)
  VbINP_HWA_FLDoorOutButton_flg_VbINP_HWA_FLDoorOutButton_flg_read/1 -> REL/16(VbINP_HWA_FLDoorOutButton_flg)
  VeOUT_DHM_BDCLeReDoorHndSts_sig_VeOUT_DHM_BDCLeReDoorHndSts_sig_read/1 -> REL/45(VeOUT_DHM_BDCLeReDoorHndSts_sig)
  VeOUT_DHM_BDCRiReDoorHndSts_sig_VeOUT_DHM_BDCRiReDoorHndSts_sig_read/1 -> REL/46(VeOUT_DHM_BDCRiReDoorHndSts_sig)
  VbINP_HWA_LRChildLckSt_flg_VbINP_HWA_LRChildLckSt_flg_read/1 -> REL/13(VbINP_HWA_LRChildLckSt_flg)
  VbINP_HWA_RRChildLckSt_flg_VbINP_HWA_RRChildLckSt_flg_read/1 -> REL/14(VbINP_HWA_RRChildLckSt_flg)
  VbOUT_SP_CrashOutpSts_flg_VbOUT_SP_CrashOutpSts_flg_read/1 -> REL/47(VbOUT_SP_CrashOutpSts_flg)
  VmOUT_DLK_LockSrc_enum_VmOUT_DLK_LockSrc_enum_read/1 -> REL/12(VmOUT_DLK_LockSrc_enum)
  VbINP_HWA_RLDoorButton_flg_VbINP_HWA_RLDoorButton_flg_read/1 -> REL/10(VbINP_HWA_RLDoorButton_flg)
  VbINP_HWA_RRDoorButton_flg_VbINP_HWA_RRDoorButton_flg_read/1 -> REL/11(VbINP_HWA_RRDoorButton_flg)
  VbINP_HWA_FLDoorButton_flg_VbINP_HWA_FLDoorButton_flg_read/1 -> REL/8(VbINP_HWA_FLDoorButton_flg)
  VbINP_HWA_FRDoorButton_flg_VbINP_HWA_FRDoorButton_flg_read/1 -> REL/9(VbINP_HWA_FRDoorButton_flg)
  VeINP_CAN_VcuGearPosn_sig_VeINP_CAN_VcuGearPosn_sig_read/1 -> REL/7(VeINP_CAN_VcuGearPosn_sig)
  VeOUT_SP_EspVehSpd_kmh_VeOUT_SP_EspVehSpd_kmh_read/1 -> REL/5(VeOUT_SP_EspVehSpd_kmh)
  VbINP_CAN_EspVehSpdVld_flg_VbINP_CAN_EspVehSpdVld_flg_read/1 -> REL/6(VbINP_CAN_EspVehSpdVld_flg)
  VeINP_EPRM_BdcDrvrDoorLockSetSts_sig_VeINP_EPRM_BdcDrvrDoorLockSetSts_sig_read/1 -> REL/3(VeINP_EPRM_BdcDrvrDoorLockSetSts_sig)
  VeOUT_DLK_BdcDrvrDoorLockSts_sig_VeOUT_DLK_BdcDrvrDoorLockSts_sig_read/1 -> REL/4(VeOUT_DLK_BdcDrvrDoorLockSts_sig)
  VeINP_CAN_CdcDrvrDoorLockSet_sig_VeINP_CAN_CdcDrvrDoorLockSet_sig_read/1 -> REL/2(VeINP_CAN_CdcDrvrDoorLockSet_sig)
  VeOUT_PDU_BcmPowerStatusFeedback_sig_VeOUT_PDU_BcmPowerStatusFeedback_sig_read/1 -> REL/1(VeOUT_PDU_BcmPowerStatusFeedback_sig)
